simulink model "Wireless_networking_fm_receiver"  (R2017b)
settings: Solver=VariableStepAuto  StartTime=0.0  StopTime=inf  RelTol=1e-3
undefined symbols (not defined in the file): designMultirateFIR
libraries: dspmlti4 x2, dspsnks4 x1, rtlsdr_book_library x1, sdrrlib x1
settings Model: Creator=Kevin  LastModifiedBy=Kevin

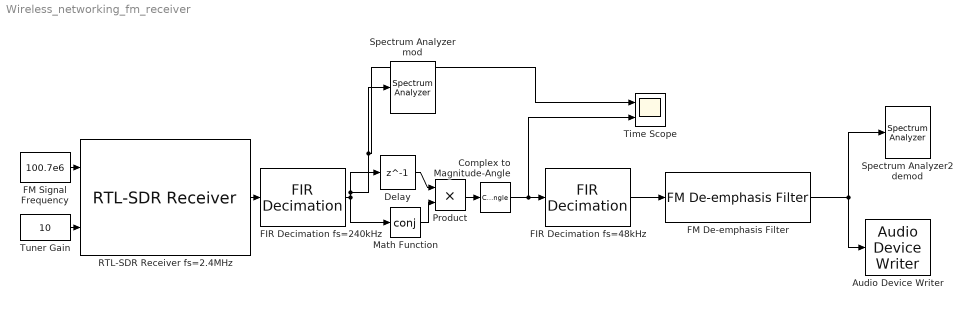
== system Wireless_networking_fm_receiver ==
  Audio Device Writer : dspsnks4/Audio Device Writer  Driver=DirectSound  Device=Speakers / Headphones (Realtek Audio)  InheritSampleRate=on  SampleRate=44100  BitDepth=16-bit integer  BufferSize=4096  NumBuffers=10  DefaultOutputChannelMapping=on  OutputChannelMapping=1:2  OutputNumUnderrunSamples=off  DriverIdx=1  DeviceWarnFlag=''
  Complex to Magnitude-Angle : ComplexToMagnitudeAngle  Output=Angle
  Delay : Delay  DelayLength=1  InputProcessing=Columns as channels (frame based)
  FIR Decimation fs=240kHz : dspmlti4/FIR Decimation  FilterSource=Auto  h=designMultirateFIR(1,2)  D=10  filtStruct=Direct form  FilterObject=FDECIM  InputProcessing=Columns as channels (frame based)  framing=Allow multirate processing  inputOffset=0  outputBufInitCond=0  roundingMode=Floor  overflowMode=off  firstCoeffDataTypeStr=Inherit: Same word length as input  firstCoeffMin=[]  firstCoeffMax=[]  firstCoeffLastDataTypeStr=Inherit: Same word length as input  outputDataTypeStr=Inherit: Same as accumulator  outputMin=[]  outputMax=[]  outputLastDataTypeStr=Inherit: Same as accumulator
  FIR Decimation fs=48kHz : dspmlti4/FIR Decimation  FilterSource=Dialog parameters  h=firpm(100, [0 53e3 60e3 (240e3/2)]/(240e3/2), [1 1 0 0], [1 1],20)  D=5  filtStruct=Direct form  FilterObject=FDECIM  InputProcessing=Columns as channels (frame based)  framing=Allow multirate processing  inputOffset=0  outputBufInitCond=0  roundingMode=Floor  overflowMode=off  firstCoeffDataTypeStr=Inherit: Same word length as input  firstCoeffMin=[]  firstCoeffMax=[]  firstCoeffLastDataTypeStr=Inherit: Same word length as input  outputDataTypeStr=Inherit: Same as accumulator  outputMin=[]  outputMax=[]  outputLastDataTypeStr=Inherit: Same as accumulator
  FM De-emphasis Filter : rtlsdr_book_library/FM Demod Tools/FM De-emphasis Filter  region=Europe, Asia  fs=48e3
      settings: SourceProductName=RTL-SDR Book Library
  FM Signal Frequency : Constant  Value=100.7e6
  Math Function : Math  Operator=conj  SaturateOnIntegerOverflow=on
  Product : Product
  RTL-SDR Receiver fs=2.4MHz : sdrrlib/RTL-SDR Receiver  SourceLibraryInfo="This block requires <a href=\"http://www.mathworks.com/hardware-support/rtl-sdr.html\">Communications System Toolbox Support Package for RTL-SDR Radio</a>"  IPAddress=0  CenterFrequencySource=Input port  CenterFrequency=97.1e6  GainSource=Input port  Gain=0  ADCRate=2.4e6  FrequencyCorrection=0  LostSamplesOutputPort=off  LatencyOutputPort=off  OutputDataType=single  FrameLength=4096  EnableBurstMode=off  NumFramesInBurst=20  sobjType=sdrr.internal.SDRRTLReceiverSL  dataUDPPort=-1  ctrlUDPPort=-1  subDeviceList=nosubdev  sdrBlockType=SDRBlockTypeSLT.SDRRxBlock  requester=UNUSED_BY_SFCN  sdrExecutionMode=SDRExecutionModeSLT.ExecModeHW  BypassUserLogic=off  DecimatorSelect=DDC decimator  SourceSelect=RF data  SineAmplitude=16000  EnableInternalClock=off  BypassIQBalance=off  IFBandwidth=40e6  ADCRateSource=Dialog  IntermediateFrequency=0  DecimationFactorSource=Dialog  DecimationFactor=512  RFFrequencyIsTunable=logical(1)  SampleTime=(4096)/(2.4e6)  IFBandwidthSource=Dialog  SineFrequency=30000  BypassDCBlockingFilter=off  IntermediateFrequencySource=Dialog  IQBalanceCoefficients=64  SkipAllHardwareResetAndInitialization=off  EnableIQCalibrationTable=on  CacheIQCalibrationTable=off  EnableOffsetTuning=off  EnableRTLAGC=off  EnableTestMode=off  EnableTunerAGC=on  FrequencyCorrectionSource=Dialog  NumMLBuffers=128  NumUSBBuffers=16  RTLCrystalFrequency=28800000  TunerCrystalFrequency=28800000
      settings: SourceProductName=Communications System Toolbox Support Package for RTL-SDR Radio  SourceProductBaseCode=RTLSDR
  Spectrum Analyzer mod : SpectrumAnalyzer
  "Spectrum Analyzer2 demod " : SpectrumAnalyzer
  Time Scope : Scope  NumInputPorts=2
  Tuner Gain : Constant  Value=10
  wires:
  FM Signal Frequency/1 -> RTL-SDR Receiver fs=2.4MHz/1
  Tuner Gain/1 -> RTL-SDR Receiver fs=2.4MHz/2
  RTL-SDR Receiver fs=2.4MHz/1 -> FIR Decimation fs=240kHz/1
  FIR Decimation fs=240kHz/1 -> Math Function/1, Time Scope/1, Spectrum Analyzer mod/1, Delay/1
  Delay/1 -> Product/1
  Math Function/1 -> Product/2
  Product/1 -> Complex to Magnitude-Angle/1
  Complex to Magnitude-Angle/1 -> Time Scope/2, FIR Decimation fs=48kHz/1
  FIR Decimation fs=48kHz/1 -> FM De-emphasis Filter/1
  FM De-emphasis Filter/1 -> Audio Device Writer/1, "Spectrum Analyzer2 demod "/1
